simulink model "aie_hls"  (R2019b)
settings: Solver=VariableStepAuto  StartTime=0.0  StopTime=4000  RelTol=1e-3
InitFcn:
  | xmcCheckSlxPath(bdroot);
  | input = readcomplexdata('./sw/input.h');
undefined symbols (not defined in the file or in its folder): xc7vx485tffg1157
libraries: ModelComposer x6, dspsrcs4 x1
settings Model: Creator=abehbood  LastModifiedBy=abehbood
settings SFSimCC: CustomCodeUndefinedFunction=UseInterfaceOnly

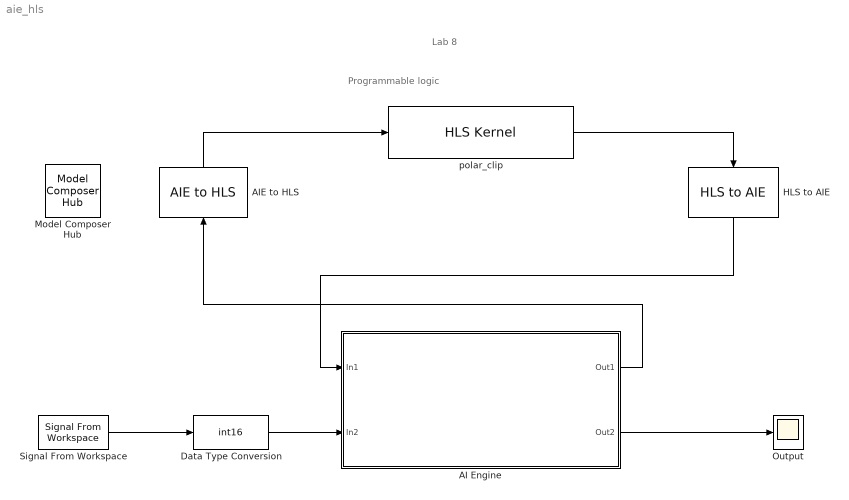
== system aie_hls ==
  note: Lab 8
  note: Programmable logic
  AI Engine : Subsystem
  AIE to HLS : ModelComposer/AIE to HLS  OutputType=ap_axis<32,0,0,0>  OutputSize=256
  Data Type Conversion : DataTypeConversion  OutDataTypeStr=int16
  HLS to AIE : ModelComposer/HLS to AIE  OutputType=cint16  OutputSize=256
  Model Composer Hub : ModelComposer/Model Composer Hub  CodeGeneration=off  SubsystemName=AI Engine  TargetDirectory=./code  ExportType=AI Engines  IpVendor=xilinx.com  IpLibrary=hls  IpVersion=1.0  IpHWLanguage=Verilog  AieCompilerOptions={}  CreateTestbench=on  TestbenchStackSize=10  RunAieSim=on  AieSimTimeout=150000  LaunchVitisAnalyzer=off  RunX86Sim=off  X86SimTimeout=10  ProjDevice=xc7vx485tffg1157-1  ProjDevicePart=xc7vx485tffg1157-1  SamplePeriod=-1  ClockFrequency=200  DataPathParallelism=1
  Output : Scope
  Signal From Workspace : dspsrcs4/Signal From Workspace  X=input  Ts=1  nsamps=128  OutputAfterFinalValue=Setting to zero  ignoreOrWarnInputAndFrameLengths=off  OutputFrames=off
  polar_clip : ModelComposer/HLS Kernel  PortAttributesTable={ 'Input', 'in_sample', 'adf::dir::in< hls::stream< hls::axis< ap_int< 32 >, 0, 0, 0 >, 0 > & >', '', ''; 'Output', 'out_sample', 'adf::dir::out< hls::stream< hls::axis< ap_int< 32 >, 0, 0, 0 >, 0 > & >', '', '256' }  PortAttributesEnablement={'off', 'off', 'off', 'off', 'off';'off', 'off', 'off', 'off', 'on'}  FormalArgDecls={'adf::dir::in< hls::stream< hls::axis< ap_int< 32 >, 0, 0, 0 >, 0 > & > in_sample', 'adf::dir::out< hls::stream< hls::axis< ap_int< 32 >, 0, 0, 0 >, 0 > & > out_sample'}  PortSynchronicities={'auto'; 'auto'}  PortSignalSizes={0.000000000000000000e+00; 2.560000000000000000e+02}  SimLibPath=''  FunctionTabVisible=on  FunctionDescription=void polar_clip(adf::dir::in< hls::stream< hls::axis< ap_int< 32 >, 0, 0, 0 >, 0 > & > in_sample, adf::dir::out< hls::stream< hls::axis< ap_int< 32 >, 0, 0, 0 >, 0 > & > out_sample)  KernelHeaderFile=src/hls_kernels.h  KernelFunction=polar_clip  KernelFunctionSelect=<empty>  KernelSourceFile=src/polar_clip.cpp  KernelSearchPaths={}  PreProcOptions={}
  wires:
  polar_clip/1 -> HLS to AIE/1
  Signal From Workspace/1 -> Data Type Conversion/1
  AIE to HLS/1 -> polar_clip/1
  HLS to AIE/1 -> AI Engine/1(In1)
  Data Type Conversion/1 -> AI Engine/2(In2)
  AI Engine/1(Out1) -> AIE to HLS/1
  AI Engine/2(Out2) -> Output/1

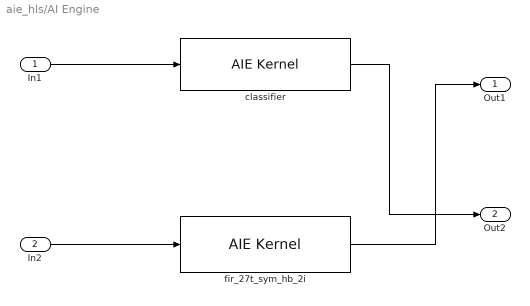
== system aie_hls/AI Engine ==
  In1 : Inport
  In2 : Inport  Port=2
  classifier : ModelComposer/AIE Kernel  PortAttributesTable={ 'Input', 'input', 'input_stream_cint16 *', '', '', '', ''; 'Output', 'output', 'output_window_int32 *', '256', '', 'sync', '' }  PortAttributesEnablement={'off', 'off', 'off', 'off', 'off', 'off', 'off';'off', 'off', 'off', 'on', 'off', 'on', 'off'}  FormalArgDecls={'input_stream_cint16 * input', 'output_window_int32 * output'}  PortWindowSizes={0.000000000000000000e+00, 2.560000000000000000e+02}  PortWindowMargins={0.000000000000000000e+00, 0.000000000000000000e+00}  PortSynchronicities={'sync', 'sync'}  PortSignalSizes={0.000000000000000000e+00, 0.000000000000000000e+00}  SimLibPath=''  FunctionTabVisible=on  FunctionDescription=void classifier(input_stream_cint16 * input, output_window_int32 * output)  KernelHeaderFile=src/kernels.h  KernelFunction=classifier  KernelFunctionSelect=<empty>  KernelSourceFile=src/kernels/classifiers/classify.cc  KernelSearchPaths={}  PreProcOptions={}  CoreRuntimeRatio=0.9
  fir_27t_sym_hb_2i : ModelComposer/AIE Kernel  PortAttributesTable={ 'Input', 'inputcb', 'input_window_cint16 *', '128', '16', 'sync', ''; 'Output', 'outputcb', 'output_window_cint16 *', '256', '', 'sync', '' }  PortAttributesEnablement={'off', 'off', 'off', 'on', 'on', 'on', 'off';'off', 'off', 'off', 'on', 'off', 'on', 'off'}  FormalArgDecls={'input_window_cint16 * inputcb', 'output_window_cint16 * outputcb'}  PortWindowSizes={1.280000000000000000e+02, 2.560000000000000000e+02}  PortWindowMargins={1.600000000000000000e+01, 0.000000000000000000e+00}  PortSynchronicities={'sync', 'sync'}  PortSignalSizes={0.000000000000000000e+00, 0.000000000000000000e+00}  SimLibPath=''  FunctionTabVisible=on  FunctionDescription=void fir_27t_sym_hb_2i(input_window_cint16 * inputcb, output_window_cint16 * outputcb)  KernelHeaderFile=src/kernels.h  KernelFunction=fir_27t_sym_hb_2i  KernelFunctionSelect=<empty>  KernelSourceFile=src/kernels/interpolators/hb27_2i.cc  KernelSearchPaths={}  PreProcOptions={}  CoreRuntimeRatio=0.9
  Out1 : Outport  VectorParamsAs1DForOutWhenUnconnected=off
  Out2 : Outport  Port=2  VectorParamsAs1DForOutWhenUnconnected=off
  wires:
  In1/1 -> classifier/1
  In2/1 -> fir_27t_sym_hb_2i/1
  classifier/1 -> Out2/1
  fir_27t_sym_hb_2i/1 -> Out1/1
